simulink model "vehicle_plant"  (R2022a)
settings: Solver=VariableStepAuto  StartTime=0.0  StopTime=30  RelTol=1e-3
undefined symbols (not defined in the file): A, Af, B, C, Cd, D, f, g, m, rho
settings Model: Creator=joseg  LastModifiedBy=maria
settings ModelReferenceCC: EnableRefExpFcnMdlSchedulingChecks=off
settings RTWCC: Description=Generic Real-Time Target

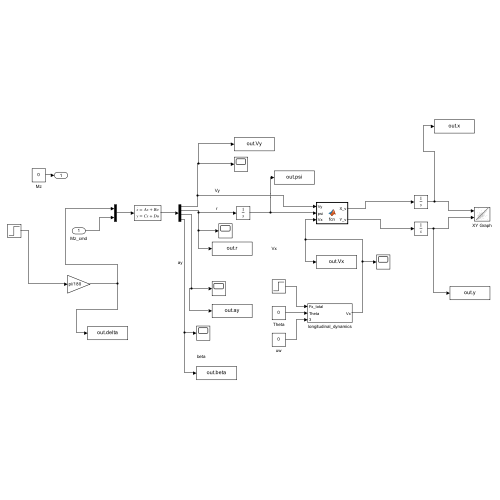
[thumbnail: Simulink's stored preview of the top-level diagram]
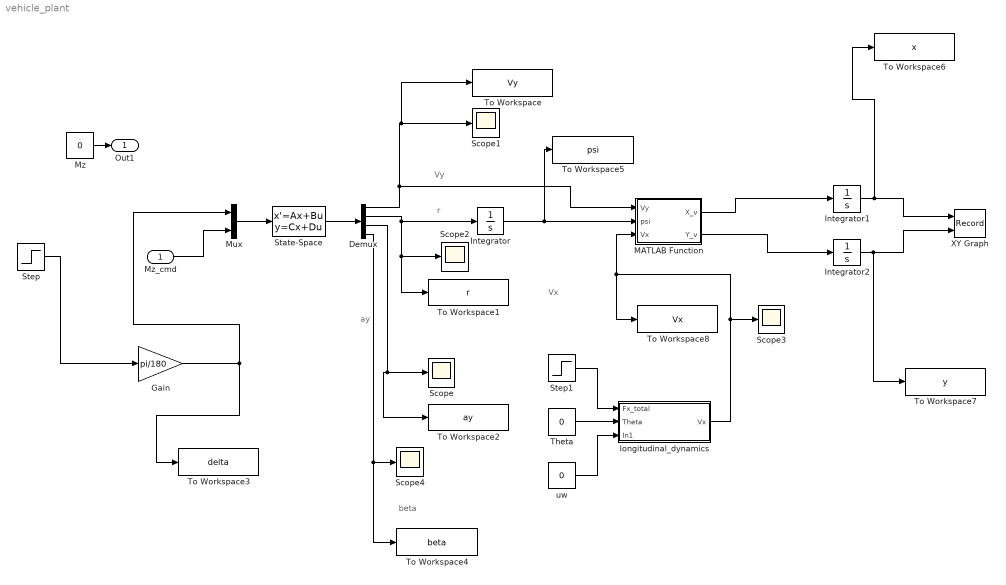
== system vehicle_plant ==
  note: ay
  note: Vx
  note: Vy
  note: r
  note: beta
  Mz_cmd : Inport
  Demux : Demux
  Gain : Gain  Gain=pi/180
  Integrator : Integrator
  Integrator1 : Integrator
  Integrator2 : Integrator
  MATLAB Function : MATLAB Function  TreatAsAtomicUnit=on
  Mux : Mux  Inputs=2
  Mz : Constant  Value=0
  Scope{,1..4} (5 alike) : Scope
  State-Space : StateSpace  A=A  B=B  C=C  D=D  InitialCondition=[0;0]
  Step : Step  After=10  SampleTime=0
  Step1 : Step  Before=461  After=461  SampleTime=0
  Theta : Constant  Value=0
  To Workspace : ToWorkspace  VariableName=Vy  SampleTime=-1
      settings: Save2DSignal=2-D array (concatenate along first dimension)
  To Workspace1 : ToWorkspace  VariableName=r  SampleTime=-1
      settings: Save2DSignal=2-D array (concatenate along first dimension)
  To Workspace2 : ToWorkspace  VariableName=ay  SampleTime=-1
      settings: Save2DSignal=2-D array (concatenate along first dimension)
  To Workspace3 : ToWorkspace  VariableName=delta  SampleTime=-1
      settings: Save2DSignal=2-D array (concatenate along first dimension)
  To Workspace4 : ToWorkspace  VariableName=beta  SampleTime=-1
      settings: Save2DSignal=2-D array (concatenate along first dimension)
  To Workspace5 : ToWorkspace  VariableName=psi  SampleTime=-1
      settings: Save2DSignal=2-D array (concatenate along first dimension)
  To Workspace6 : ToWorkspace  VariableName=x  SampleTime=-1
      settings: Save2DSignal=2-D array (concatenate along first dimension)
  To Workspace7 : ToWorkspace  VariableName=y  SampleTime=-1
      settings: Save2DSignal=2-D array (concatenate along first dimension)
  To Workspace8 : ToWorkspace  VariableName=Vx  SampleTime=-1
      settings: Save2DSignal=2-D array (concatenate along first dimension)
  XY Graph : Record  FileSettingsInternal="{\"entries\":[{\"content\":{\"excelSettings\":{\"content\":{},\"type\":\"Streamout.ExcelSettings\"}},\"type\":\"Streamout.FileSettingStorage\",\"uuid\":\"\"}],\"packageUris\":[\"http:\\/\\/schema.mathworks.com\\/mf0\\/streamout_blocks\\/R2020a\"],\"version\":\"1.0\"}"  Layout=[1 1]  SignalsInternal="{\"entries\":[{\"content\":{\"signals\":[{\"content\":{\"blockPath\":[],\"dimensions\":[1],\"domain\":\"\",\"lineColor\":\"#a2142f\",\"plots\":[ 1 ],\"port\":1,\"signalID\":1,\"signalName\":\"Integrator1\"},\"type\":\"RecordBlkView.Signal\",\"uuid\":\"\"},{\"content\":{\"blockPath\":[],\"dimensions\":[1],\"domain\":\"\",\"lineColor\":\"#ff13a6\",\"lineWidth\":2,\"port\":1,\"signalID\":2,\"signalName\":\"Demux:1\"},\"type\":\"RecordBlkView.Signal\",\"uuid\":\"\"},{\"content\":{\"blockPath\":[],\"dimensions\":[1],\"domain\":\"\",\"lineColor\":\"#fe330a\",\"lineWidth\":2,\"port\":1,\"signalID\":3,\"signalName\":\"Demux:2\"},\"type\":\"RecordBlkView.Signal\",\"uuid\":\"\"},{\"content\":{\"blockPath\":[],\"dimensions\":[1],\"domain\":\"\",\"lineColor\":\"#22b573\",\"lineWidth\":2,\"port\":1,\"signalID\":4,\"signalName\":\"Demux:3\"},\"type\":\"RecordBlkView.Signal\",\"uuid\":\"\"},{\"content\":{\"blockPath\":[],\"dimensions\":[1],\"domain\":\"\",\"lineColor\":\"#0072bd\",\"lineWidth\":2,\"port\":1,\"signalID\":5,\"signalName\":\"Gain\"},\"type\":\"RecordBlkView.Signal\",\"uuid\":\"\"},{\"content\":{\"blockPath\":[],\"dimensions\":[1],\"domain\":\"\",\"lineColor\":\"#d95319\",\"lineWidth\":2,\"port\":1,\"signalID\":6,\"signalName\":\"Demux:4\"},\"type\":\"RecordBlkView.Signal\",\"uuid\":\"\"},{\"content\":{\"blockPath\":[],\"dimensions\":[1],\"domain\":\"\",\"lineColor\":\"#edb120\",\"lineWidth\":2,\"port\":1,\"signalID\":7,\"signalName\":\"Integrator\"},\"type\":\"RecordBlkView.Signal\",\"uuid\":\"\"},{\"content\":{\"blockPath\":[],\"dimensions\":[1],\"domain\":\"\",\"lineColor\":\"#7e2f8e\",\"lineWidth\":2,\"port\":1,\"signalID\":8,\"signalName\":\"Integrator1\"},\"type\":\"RecordBlkView.Signal\",\"uuid\":\"\"},{\"content\":{\"blockPath\":[],\"dimensions\":[1],\"domain\":\"\",\"lineColor\":\"#77ac30\",\"lineWidth\":2,\"port\":1,\"signalID\":9,\"signalName\":\"Integrator2\"},\"type\":\"RecordBlkView.Signal\",\"uuid\":\"\"},{\"content\":{\"blockPath\":[],\"dimensions\":[1],\"domain\":\"\",\"lineColor\":\"#a2142f\",\"lineWidth\":2,\"port\":1,\"signalID\":10,\"signalName\":\"longitudinal_dynamics\"},\"type\":\"RecordBlkView.Signal\",\"uuid\":\"\"},{\"content\":{\"blockPath\":[],\"dimensions\":[1],\"domain\":\"\",\"lineColor\":\"#4dbeee\",\"lineWidth\":2,\"port\":1,\"signalID\":11,\"signalName\":\"Fx_total\"},\"type\":\"RecordBlkView.Signal\",\"uuid\":\"\"},{\"content\":{\"blockPath\":[],\"dimensions\":[1],\"domain\":\"\",\"lineColor\":\"#139fff\",\"lineWidth\":2,\"port\":1,\"signalID\":12,\"signalName\":\"In1\"},\"type\":\"RecordBlkView.Signal\",\"uuid\":\"\"},{\"content\":{\"blockPath\":[],\"dimensions\":[1],\"domain\":\"\",\"lineColor\":\"#ff6929\",\"lineWidth\":2,\"port\":1,\"signalID\":13,\"signalName\":\"Theta\"},\"type\":\"RecordBlkView.Signal\",\"uuid\":\"\"},{\"content\":{\"blockPath\":[],\"dimensions\":[1],\"domain\":\"\",\"lineColor\":\"#139fff\",\"plots\":[ 1 ],\"port\":2,\"signalID\":14,\"signalName\":\"Integrator2\"},\"type\":\"RecordBlkView.Signal\",\"uuid\":\"\"}]},\"type\":\"RecordBlkView.InputSignals\",\"uuid\":\"\"}],\"packageUris\":[\"http:\\/\\/schema.mathworks.com\\/mf0\\/streamout_blocks\\/R2020a\"],\"version\":\"1.0\"}"  VisualizationBindings="{\"xyplotplugin\":{\"info\":[{\"series\":[{\"bindingParametersList\":[{\"parameter\":\"X-Axis\",\"signalID\":1,\"signalName\":\"Integrator1\"},{\"parameter\":\"Y-Axis\",\"signalID\":14,\"signalName\":\"Integrator2\"}],\"seriesID\":0}],\"subplotID\":1}]}}"  CompatibilityTag=XY
  longitudinal_dynamics : Subsystem
  uw : Constant  Value=0
  Out1 : Outport
  wires:
  State-Space/1 -> Demux/1
  Gain/1 -> To Workspace3/1, Mux/1
  Demux/2 -> To Workspace1/1, Scope2/1, Integrator/1
  Integrator/1 -> To Workspace5/1, MATLAB Function/2(psi)
  Demux/1 -> To Workspace/1, Scope1/1, MATLAB Function/1(Vy)
  Demux/3 -> Scope/1, To Workspace2/1
  MATLAB Function/1(X_v) -> Integrator1/1
  MATLAB Function/2(Y_v) -> Integrator2/1
  Integrator1/1 -> To Workspace6/1, XY Graph/1
  Integrator2/1 -> To Workspace7/1, XY Graph/2
  Step/1 -> Gain/1
  Mux/1 -> State-Space/1
  Demux/4 -> Scope4/1, To Workspace4/1
  Mz_cmd/1 -> Mux/2
  Step1/1 -> longitudinal_dynamics/1(Fx_total)
  Theta/1 -> longitudinal_dynamics/2(Theta)
  uw/1 -> longitudinal_dynamics/3(In1)
  longitudinal_dynamics/1(Vx) -> MATLAB Function/3(Vx), To Workspace8/1, Scope3/1
  Mz/1 -> Out1/1

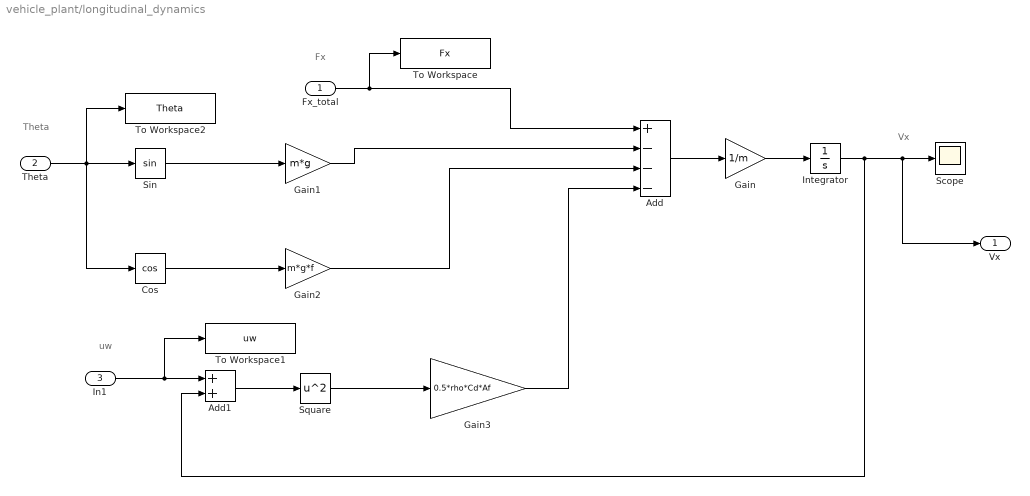
== system vehicle_plant/longitudinal_dynamics ==
  note: uw
  note: Fx
  note: Theta
  note: Vx
  Fx_total : Inport
  Theta : Inport  Port=2
  In1 : Inport  Port=3
  Add : Sum  Inputs=+---
  Add1 : Sum
  Cos : Trigonometry  Operator=cos
  Gain : Gain  Gain=1/m
  Gain1 : Gain  Gain=m*g
  Gain2 : Gain  Gain=m*g*f
  Gain3 : Gain  Gain=0.5*rho*Cd*Af
  Integrator : Integrator  InitialCondition=16
  Scope : Scope
  Sin : Trigonometry
  Square : Math  Operator=square
  To Workspace : ToWorkspace  VariableName=Fx  SampleTime=-1
      settings: Save2DSignal=2-D array (concatenate along first dimension)
  To Workspace1 : ToWorkspace  VariableName=uw  SampleTime=-1
      settings: Save2DSignal=2-D array (concatenate along first dimension)
  To Workspace2 : ToWorkspace  VariableName=Theta  SampleTime=-1
      settings: Save2DSignal=2-D array (concatenate along first dimension)
  Vx : Outport
  wires:
  Gain1/1 -> Add/2
  Add1/1 -> Square/1
  Add/1 -> Gain/1
  Gain2/1 -> Add/3
  Cos/1 -> Gain2/1
  Square/1 -> Gain3/1
  Gain/1 -> Integrator/1
  In1/1 -> To Workspace1/1, Add1/1
  Theta/1 -> To Workspace2/1, Cos/1, Sin/1
  Sin/1 -> Gain1/1
  Gain3/1 -> Add/4
  Fx_total/1 -> To Workspace/1, Add/1
  Integrator/1 -> Add1/2, Vx/1, Scope/1

== matlab function vehicle_plant/MATLAB Function ==
  data: Vy input; X_v output; psi input; Vx input; Y_v output
function [X_v, Y_v] = fcn(Vy, psi, Vx)

X_v = Vx*cos(psi) - Vy*sin(psi);
Y_v = Vx*sin(psi) + Vy*cos(psi);

end
